simulink model "Assignment_2 (1)"  (R2013a)
settings: Solver=ode45  StartTime=0.0  StopTime=6e-5  RelTol=1e-3
libraries: powerlib x11
settings Model: Creator=SUJIT  LastModifiedBy=SUJIT

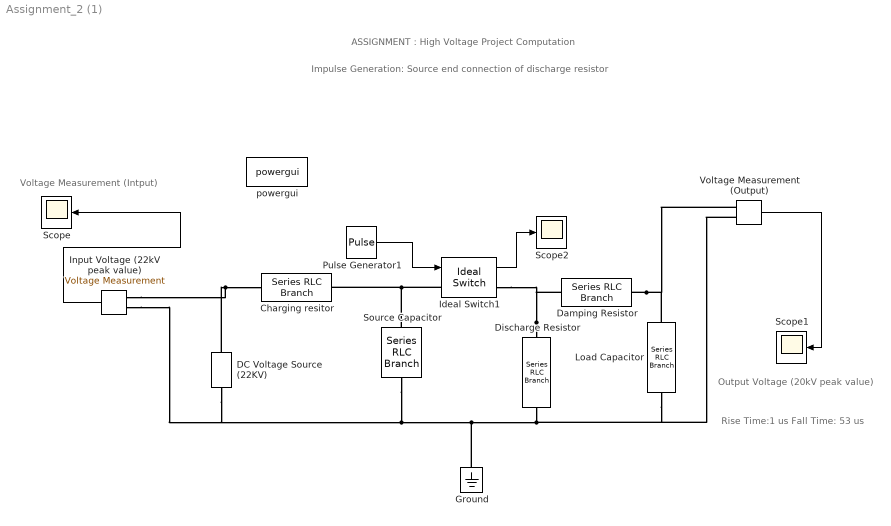
== system Assignment_2 (1) ==
  note: Rise Time:1 us
      | Fall Time: 53 us
  note: Voltage Measurement
      | 	(Intput)
  note: Output Voltage
      | (20kV peak value)
  note: Impulse Generation: Source end connection of discharge resistor
  note: ASSIGNMENT : High Voltage Project Computation
  Charging resitor : powerlib/Elements/Series RLC Branch  LConnTagsString=__new0  RConnTagsString=__new0  BranchType=R  Resistance=0.001  Inductance=1e-5  SetiL0=off  InitialCurrent=0  Capacitance=1e-6  Setx0=off  InitialVoltage=0  Measurements=None
  DC Voltage Source (22KV) : powerlib/Electrical Sources/DC Voltage Source  Amplitude=20000  Measurements=None
  Damping Resistor : powerlib/Elements/Series RLC Branch  LConnTagsString=__new0  RConnTagsString=__new0  BranchType=R  Resistance=10/6  Inductance=1e-6  SetiL0=off  InitialCurrent=0  Capacitance=1e-7  Setx0=off  InitialVoltage=0  Measurements=None
  Discharge Resistor : powerlib/Elements/Series RLC Branch  LConnTagsString=__new0  RConnTagsString=__new0  BranchType=R  Resistance=750  Inductance=1e-4  SetiL0=off  InitialCurrent=0  Capacitance=0  Setx0=off  InitialVoltage=0  Measurements=None
  Ground : powerlib/Elements/Ground  LConnTagsString=a
  Ideal Switch1 : powerlib/Power Electronics/Ideal Switch  Ron=0.0000000001  Lon=0  IC=0  Rs=1e10  Cs=inf  Measurements=on
  Input Voltage (22kV peak value) : powerlib/Measurements/Voltage Measurement  PhasorSimulation=off  OutputType=Complex  PSBequivalent=0
  Load Capacitor : powerlib/Elements/Series RLC Branch  LConnTagsString=__new0  RConnTagsString=__new0  BranchType=C  Resistance=0.00001  Inductance=1e-6  SetiL0=off  InitialCurrent=0  Capacitance=1e-7  Setx0=off  InitialVoltage=0  Measurements=None
  Pulse Generator1 : DiscretePulseGenerator  PulseType=Time based  Period=1e-4
  Scope : Scope
      settings: YMin=-1.97626e-323  YMax=4.75e-307
  Scope1 : Scope
      settings: YMin=17.7256  YMax=17.7256  MaxDataPoints=500000
  Scope2 : Scope
      settings: YMin=-1.97626e-323  YMax=4.75e-307  SaveName=ScopeData2
  Source Capacitor : powerlib/Elements/Series RLC Branch  LConnTagsString=__new0  RConnTagsString=__new0  BranchType=C  Resistance=0.0001  Inductance=1  SetiL0=off  InitialCurrent=0  Capacitance=6e-7  Setx0=off  InitialVoltage=18000  Measurements=None
  Voltage Measurement (Output) : powerlib/Measurements/Voltage Measurement  PhasorSimulation=off  OutputType=Complex  PSBequivalent=0
  powergui : powerlib/powergui  Priority=1  SimulationMode=Continuous  SolverType=Backward Euler  SampleTime=10e-7  frequency=60  SPID=off  DisableSnubberDevices=off  DisableRonSwitches=off  DisableVfSwitches=off  SwTol=0  Interpol=off  DisplayEquations=off  frequencyindice=0  Pbase=100e6  ErrMax=1e-4  Iterations=50  UnitsV=kV  UnitsW=MW  FunctionMessages=off  echomessages=off  HookPort=off  EnableUseOfTLC=off  x0status=blocks  RestoreLinks=warning  ResistiveCurrentMeasurement=off  Frange=[0:2:500]  Ylog=off  Xlog=on  ShowGrid=off  save=off  variable=ZData  ZoomFFT=off  StartTime=0.0  cycles=1  DisplayStyle=1  fundamental=60  FreqAxis=off  MaxFrequency=1000  frequencyindicesteady=1  RmsSteady=2  display=off  Ts=0  methode=off
  wires:
  Input Voltage (22kV peak value)/1 -> Scope/1
  Voltage Measurement (Output)/1 -> Scope1/1
  Ideal Switch1/1 -> Scope2/1
  Pulse Generator1/1 -> Ideal Switch1/1
  connections:
  Discharge Resistor/LConn1 -- Ideal Switch1/RConn1 -- Damping Resistor/LConn1
  DC Voltage Source (22KV)/RConn1 -- Input Voltage (22kV peak value)/LConn1 -- Charging resitor/LConn1
  Discharge Resistor/RConn1 -- Ground/LConn1 -- Input Voltage (22kV peak value)/LConn2 -- DC Voltage Source (22KV)/LConn1 -- Source Capacitor/RConn1 -- Voltage Measurement (Output)/LConn2 -- Load Capacitor/RConn1
  Damping Resistor/RConn1 -- Load Capacitor/LConn1 -- Voltage Measurement (Output)/LConn1
  Source Capacitor/LConn1 -- Ideal Switch1/LConn1 -- Charging resitor/RConn1
